simulink model "PID"  (Simulink 9.0)
settings: Solver=VariableStepAuto  StartTime=0.0  StopTime=10.0  RelTol=1e-3
InitFcn:
  | PID_config
values from neighbouring files (symbols this model uses):
  b = 3.5077E-6    (= 3.5077e-06)    [MCC_constants.m]    (also in PID_config.m = 0.0085)
  Cr = 0    [MCC_constants.m]
  J = 3.2284E-6    (= 3.2284e-06)    [MCC_constants.m]    (also in PID_config.m = 0.28)
  K = 0.0274    [MCC_constants.m]    (also in PID_config.m = 0.5093)
  Kp = 100    [PID_config.m]
  L = 2.75E-6    (= 2.75e-06)    [MCC_constants.m]    (also in PID_config.m = 0.0016)
  R = 4    [MCC_constants.m]    (also in PID_config.m = 0.13)
settings Model: Creator=TP_EO_6  LastModifiedBy=TP_EO_6
settings DataIOCC: SaveFormat=Dataset
settings OptimizationCC: LifeSpan=auto
settings DebuggingCC: UnderspecifiedInitializationDetection=Simplified  MergeDetectMultiDrivingBlocksExec=error  SFUnexpectedBacktrackingDiag=error  SFNoUnconditionalDefaultTransitionDiag=error  SFExecutionAtInitializationDiag=warning
settings HardwareCC: ProdBitPerPointer=64  ProdBitPerSizeT=64  ProdBitPerPtrDiffT=64  ProdLargestAtomicFloat=Float  ProdIntDivRoundTo=Zero  ProdEndianess=LittleEndian  ProdWordSize=64  ProdHWDeviceType=Intel->x86-64 (Windows64)
settings ModelReferenceCC: PropagateSignalLabelsOutOfModel=on
settings CodeAppCC: StateflowObjectComments=off
settings GRTTargetCC: TargetLangStandard=C99 (ISO)
settings ConfigComp: CovMetricSettings=dwe  CovHtmlReporting=off  CovSaveCumulativeToWorkspaceVar=off  CovSaveSingleToWorkspaceVar=off  CovExternalEMLEnable=on

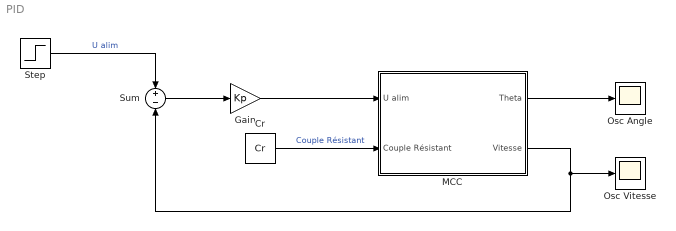
== system PID ==
  Cr : Constant  Value=Cr
  Gain : Gain  Gain=Kp
  "MCC " : Subsystem
  "Osc Angle " : Scope
  Osc Vitesse : Scope
  Step : Step  Time=0  After=12  SampleTime=0
  Sum : Sum  Inputs=+|-
  wires:
  Cr/1 -> "MCC "/2(Couple Résistant)  "Couple Résistant"
  "MCC "/1(Theta) -> "Osc Angle "/1
  Step/1 -> Sum/1  "U alim"
  Gain/1 -> "MCC "/1(U alim)
  Sum/1 -> Gain/1
  "MCC "/2(Vitesse) -> Sum/2, Osc Vitesse/1

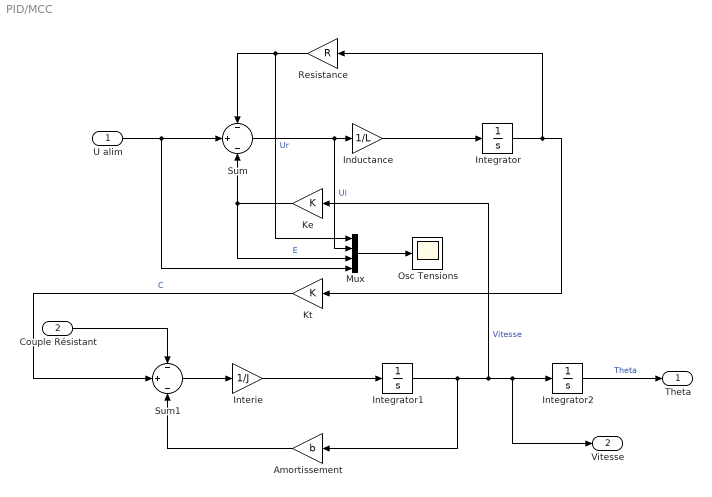
== system PID/MCC  ==
  U alim : Inport
  Couple Résistant : Inport  Port=2
  "\tInterie" : Gain  Gain=1/J
  Amortissement : Gain  Gain=b
  Inductance : Gain  Gain=1/L
  Integrator : Integrator
  Integrator1 : Integrator
  Integrator2 : Integrator
  Ke : Gain  Gain=K
  "Kt " : Gain  Gain=K
  Mux : Mux
  Osc Tensions : Scope
  Resistance : Gain  Gain=R
  Sum : Sum  Inputs=-|+|-
  Sum1 : Sum  Inputs=-|+|-
  Theta : Outport
  Vitesse : Outport  Port=2
  wires:
  Sum1/1 -> "\tInterie"/1
  Inductance/1 -> Integrator/1
  Sum/1 -> Mux/2, Inductance/1  "Ul"
  Resistance/1 -> Mux/1, Sum/1  "Ur"
  "Kt "/1 -> Sum1/2  "C"
  Ke/1 -> Sum/3, Mux/3  "E"
  Amortissement/1 -> Sum1/3
  U alim/1 -> Mux/4, Sum/2
  Mux/1 -> Osc Tensions/1
  Integrator2/1 -> Theta/1  "Theta"
  Integrator1/1 -> Amortissement/1, Ke/1, Vitesse/1, Integrator2/1  "Vitesse"
  Couple Résistant/1 -> Sum1/1
  Integrator/1 -> Resistance/1, "Kt "/1
  "\tInterie"/1 -> Integrator1/1
